simulink model "TargetModel"  (R2014a)
settings: Solver=ode3  SolverMode=SingleTasking  StartTime=0.0  StopTime=Inf  FixedStep=0.1  RelTol=1e-3
PostLoadFcn:
  | loadRobotParameters
  | 
  | allotedRunTime = 3*60; % [sec] Time allowed for run
  | 
  | % starting parameters
  | % The timer starts once the robot has moved a certain distance from the
  | % starting point
  | startPos = [50 50]; % [cm]
  | startingRadius = 10; % [cm]
  | 
  | % Target parameters
  | targetBoundaryRadius = 7; % [cm] radius considered at location
  | statTimeReq = 2.5; % [sec] minimum time robot must be at location
InitFcn:
  | close('all','force');
StartFcn:
  | %reset(SimDisplay.getInstance());
undefined symbols (not defined in the file or in its folder): AxleLength, dT, EncRes, TargetPositions, WheelRadius
libraries: arduinodue_drivers x5, simulink x3, arduinolib x2
CloseFcn:
  | close('all','force');
settings Model: SimulationMode=external  PauseTimes=14  ExtModeTrigDuration=2  Creator=gpacitti  LastModifiedBy=odufour
settings DataIOCC: SignalLoggingSaveFormat=ModelDataLogs  SaveOutput=off  SignalLogging=off  DSMLogging=off  SaveTime=off
settings OptimizationCC: ExpressionDepthLimit=2147483647  OptimizeModelRefInitCode=on  LifeSpan=Inf
settings DebuggingCC: UnderspecifiedInitializationDetection=Classic  SolverPrmCheckMsg=none  MultiTaskDSMMsg=warning  MultiTaskCondExecSysMsg=none  ParameterPrecisionLossMsg=none  StateNameClashWarn=warning
settings HardwareCC: ProdLargestAtomicInteger=Long  ProdLargestAtomicFloat=Double  ProdEndianess=LittleEndian  ProdHWDeviceType=ARM Compatible->ARM Cortex
settings RTWCC: SystemTargetFile=realtime.tlc  GenerateMakefile=off  TemplateMakefile=realtime.tmf  Description=Run on Target Hardware  RTWVerbose=off  ProcessScript=realtime_make_rtw_hook  IncludeERTFirstTime=on
settings CodeAppCC: CustomSymbolStrType=$N$R$M  InternalIdentifier=Classic
settings STFCustomTargetCC: TargetLibSuffix=.a  GenerateSampleERTMain=on  ConcurrentExecutionCompliant=off  GeneratePreprocessorConditionals=Use local settings  ERTCustomFileBanners=on  SupportNonInlinedSFcns=off  SupportVariableSizeSignals=on  MATLABClassNameForMDSCustomization=Simulink.SoftwareTarget.ERTCustomization  GRTInterface=off  SystemTargetFile=realtime.tlc
settings ERTTargetCC: CombineOutputUpdateFcns=off  SupportContinuousTime=on  SupportVariableSizeSignals=on  ExtMode=on  ExtModeTransport=3  ExtModeMexArgs=0 17 115200 30  ERTSrcFileBannerTemplate=realtime_code_template.cgt  ERTHdrFileBannerTemplate=realtime_code_template.cgt  ERTDataSrcFileTemplate=realtime_code_template.cgt  ERTDataHdrFileTemplate=realtime_code_template.cgt  ERTCustomFileTemplate=realtime_file_process.tlc
settings ConfigComp: Description=Design Verifier Custom Configuration Component  DVMaxTestCaseSteps=500  DVTestSuiteOptimization=CombinedObjectives (Nonlinear Extended)

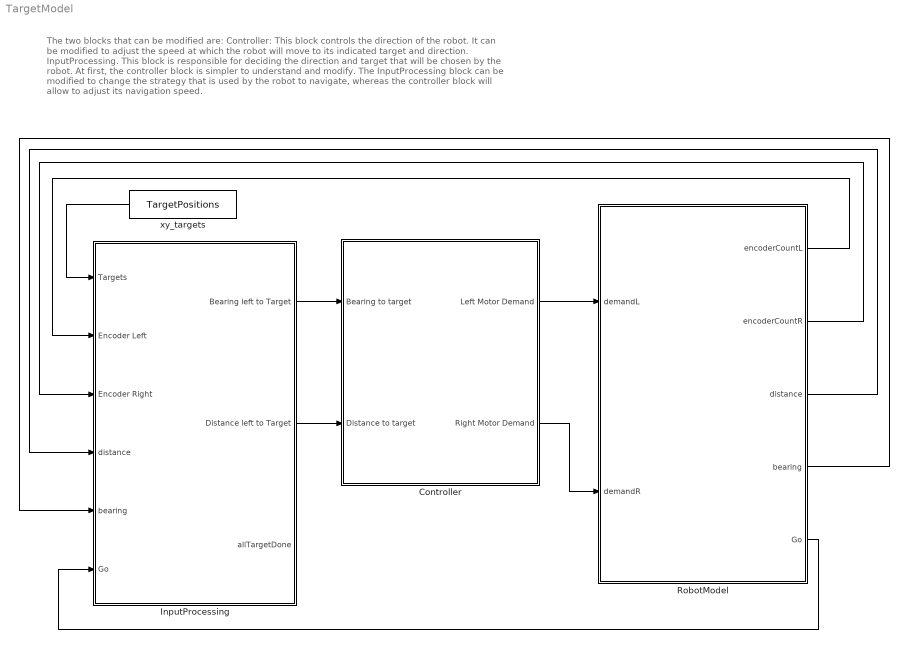
== system TargetModel ==
  note: The two blocks that can be modified are:
      | Controller: This block controls the direction of the robot. It can be modified to adjust the speed at which the robot will move to its indicated target and direction.
      | InputProcessing. This block is responsible for deciding the direction and target that will be chosen by the robot.
      |
      | At first, the controller block is simpler to understand and modify.
      | The InputProcessing block can be modified to change the strategy that is used by the robot to navigate, whereas the controller block will allow to adjust its navigation speed.
  Controller : Subsystem  TreatAsAtomicUnit=on
      mask Display: image('Arduino_Mega_2560.jpg',[0.75/2,0.3,0.25,0.4]);
  InputProcessing : Subsystem
      mask Display: image('Arduino_Mega_2560.jpg',[0.75/2,0.3,0.25,0.3]);
  RobotModel : Subsystem
      mask Display: image('robot_3d.jpg',[0.20,0.3,0.45,0.3]);
  xy_targets : Constant  Value=TargetPositions  OutDataTypeStr=single  SampleTime=1
  wires:
  RobotModel/2(encoderCountR) -> InputProcessing/3(Encoder Right)
  RobotModel/1(encoderCountL) -> InputProcessing/2(Encoder Left)
  xy_targets/1 -> InputProcessing/1(Targets)
  InputProcessing/2(Distance left to Target) -> Controller/2(Distance to target)
  InputProcessing/1(Bearing left to Target) -> Controller/1(Bearing to target)
  Controller/1(Left Motor Demand) -> RobotModel/1(demandL)
  Controller/2(Right Motor Demand) -> RobotModel/2(demandR)
  RobotModel/3(distance) -> InputProcessing/4(distance)
  RobotModel/4(bearing) -> InputProcessing/5(bearing)
  RobotModel/5(Go) -> InputProcessing/6(Go)

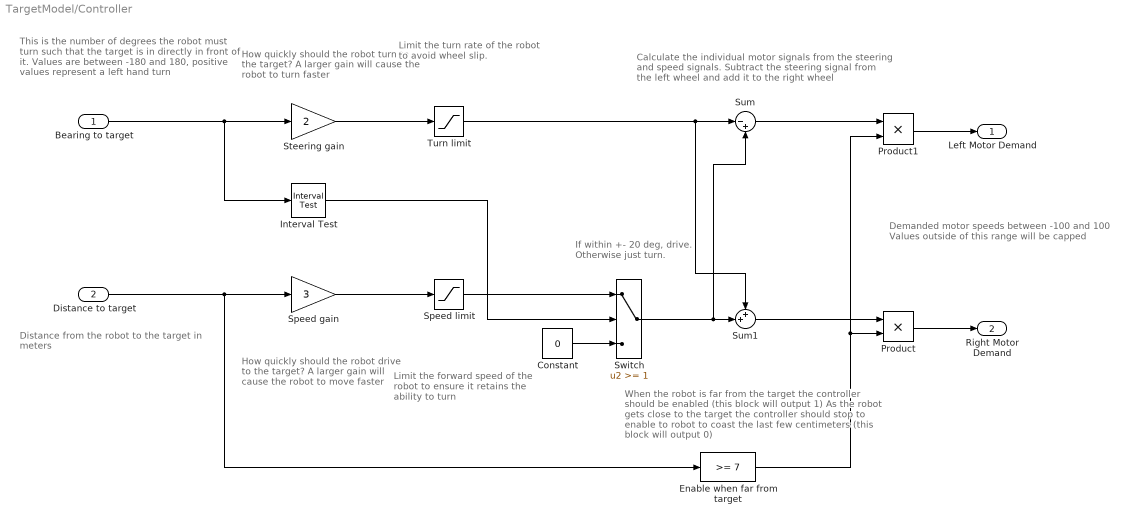
== system TargetModel/Controller ==
  note: This is the number of degrees the robot
      | must turn such that the target is in directly
      | in front of it.
      | Values are between -180 and 180,
      | positive values represent a left hand turn
  note: Distance from the robot to the target
      | in meters
  note: Demanded motor speeds between -100 and 100
      | Values outside of this range will be capped
  note: How quickly should the robot turn
      | to the target? A larger gain will
      |  cause the robot to turn faster
  note: How quickly should the robot
      | drive to the target? A larger gain
      | will cause the robot to move
      | faster
  note: Limit the forward speed of the
      | robot to ensure it retains the
      | ability to turn
  note: When the robot is far from the target the controller
      | should be enabled (this block will output 1)
      | As the robot gets close to the target the controller
      | should stop to enable to robot to coast the last
      | few centimeters (this block will output 0)
  note: Calculate the individual motor signals from the
      | steering and speed signals. Subtract the steering
      | signal from the left wheel and add it to the right
      | wheel
  note: If within +- 20 deg, drive.
      | Otherwise just turn.
  note: Limit the turn rate of the
      | robot to avoid wheel slip.
  Bearing to target : Inport  OutDataTypeStr=single
  Distance to target : Inport  Port=2  PortDimensions=1  SampleTime=dT
  Constant : Constant  Value=0  OutDataTypeStr=single
  Enable when far from target : simulink/Logic and Bit Operations/Compare To Constant  relop=>=  const=7  OutDataTypeStr=uint8
  Interval Test : simulink/Logic and Bit Operations/Interval Test  IntervalClosedRight=on  uplimit=20  IntervalClosedLeft=on  lowlimit=-20  OutDataTypeStr=boolean
      settings: AttributesFormatString=|
      | Upper = %<uplimit>
      | Lower = %<lowlimit>
  Product : Product
  Product1 : Product
  Speed gain : Gain  Gain=3
  Speed limit : Saturate  UpperLimit=40  LowerLimit=0
      settings: AttributesFormatString=|
      | Upper = %<UpperLimit>
      | Lower = %<LowerLimit>
  Steering gain : Gain  Gain=2
  Sum : Sum  Inputs=|-+
  Sum1 : Sum  Inputs=++|
  Switch : Switch  Threshold=1
  Turn limit : Saturate  UpperLimit=50  LowerLimit=-50
      settings: AttributesFormatString=|
      | Upper = %<UpperLimit>
      | Lower = %<LowerLimit>
  Left Motor Demand : Outport  OutDataTypeStr=single
  Right Motor Demand : Outport  Port=2  OutDataTypeStr=single
  wires:
  Speed limit/1 -> Switch/1
  Turn limit/1 -> Sum1/1, Sum/1
  Constant/1 -> Switch/3
  Interval Test/1 -> Switch/2
  Sum/1 -> Product1/1
  Sum1/1 -> Product/1
  Bearing to target/1 -> Steering gain/1, Interval Test/1
  Switch/1 -> Sum1/2, Sum/2
  Enable when far from target/1 -> Product1/2, Product/2
  Product1/1 -> Left Motor Demand/1
  Product/1 -> Right Motor Demand/1
  Speed gain/1 -> Speed limit/1
  Steering gain/1 -> Turn limit/1
  Distance to target/1 -> Enable when far from target/1, Speed gain/1

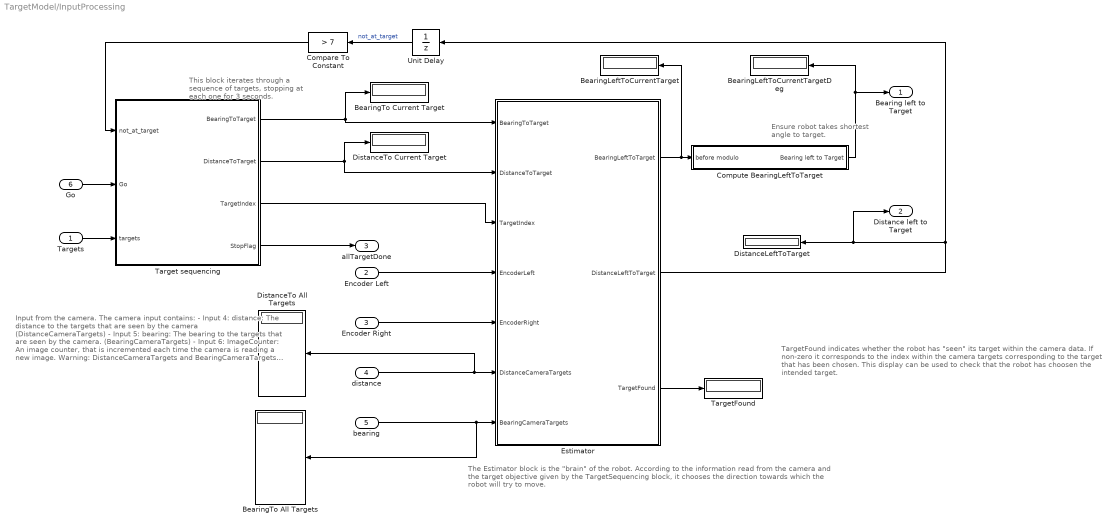
== system TargetModel/InputProcessing ==
  note: TargetFound indicates whether the robot has "seen" its target within the camera
      | data.
      | If non-zero it corresponds to the index within the camera targets corresponding
      | to the target that has been chosen.
      |
      | This display can be used to check that the robot has choosen the intended
      | target.
  note: The Estimator block is the "brain" of the robot. According to the information read from the camera and the
      | target objective given by the TargetSequencing block, it chooses the direction towards which the robot
      | will try to move.
  note: Ensure robot takes shortest
      | angle to target.
  note: This block iterates through a
      | sequence of targets, stopping
      | at each one for 3 seconds.
  note: Input from the camera. The camera input contains:
      | - Input 4: distance: The distance to the targets that are seen by the
      |   camera (DistanceCameraTargets)
      | - Input 5: bearing: The bearing to the targets that are seen
      |   by the camera. (BearingCameraTargets)
      | - Input 6: ImageCounter: An image counter, that is incremented
      |   each time the camera is reading a new image.
      | Warning: DistanceCameraTargets and BearingCameraTargets
      | are the targets seen by the camera. So for instance, the
      | target 1 is the first target seen by the camera, but is not the
      | same target as the target at index 1 within the target sequencing
      | block.
  Targets : Inport
  Encoder Left : Inport  Port=2  OutDataTypeStr=class(intEncoder(0))
  Encoder Right : Inport  Port=3  OutDataTypeStr=class(intEncoder(0))
  distance : Inport  Port=4
  bearing : Inport  Port=5
  Go : Inport  Port=6
  BearingLeftToCurrentTarget : Display
  BearingLeftToCurrentTargetDeg : Display
  BearingTo All Targets : Display
  "BearingTo Current Target " : Display
  Compare To Constant : simulink/Logic and Bit Operations/Compare To Constant  relop=>  const=7  OutDataTypeStr=boolean
  Compute BearingLeftToTarget : Subsystem
  DistanceLeftToTarget : Display
  DistanceTo All Targets : Display
  DistanceTo Current Target : Display
  Estimator : MATLAB Function  TreatAsAtomicUnit=on
  Target sequencing : MATLAB Function  TreatAsAtomicUnit=on  SystemSampleTime=dT
  TargetFound : Display
  Unit Delay : UnitDelay  SampleTime=dT
  Bearing left to Target : Outport  SampleTime=dT
  Distance left to Target : Outport  Port=2
  allTargetDone : Outport  Port=3
  wires:
  Go/1 -> Target sequencing/2(Go)
  distance/1 -> DistanceTo All Targets/1, Estimator/6(DistanceCameraTargets)
  bearing/1 -> Estimator/7(BearingCameraTargets), BearingTo All Targets/1
  Target sequencing/4(StopFlag) -> allTargetDone/1
  Compare To Constant/1 -> Target sequencing/1(not_at_target)
  Compute BearingLeftToTarget/1(Bearing left to Target) -> BearingLeftToCurrentTargetDeg/1, Bearing left to Target/1
  Estimator/3(TargetFound) -> TargetFound/1
  Target sequencing/3(TargetIndex) -> Estimator/3(TargetIndex)
  Estimator/2(DistanceLeftToTarget) -> DistanceLeftToTarget/1, Distance left to Target/1, Unit Delay/1
  Estimator/1(BearingLeftToTarget) -> BearingLeftToCurrentTarget/1, Compute BearingLeftToTarget/1(before modulo)
  Target sequencing/1(BearingToTarget) -> Estimator/1(BearingToTarget), "BearingTo Current Target "/1
  Unit Delay/1 -> Compare To Constant/1  "not_at_target"
  Encoder Right/1 -> Estimator/5(EncoderRight)
  Target sequencing/2(DistanceToTarget) -> Estimator/2(DistanceToTarget), DistanceTo Current Target/1
  Encoder Left/1 -> Estimator/4(EncoderLeft)
  Targets/1 -> Target sequencing/3(targets)

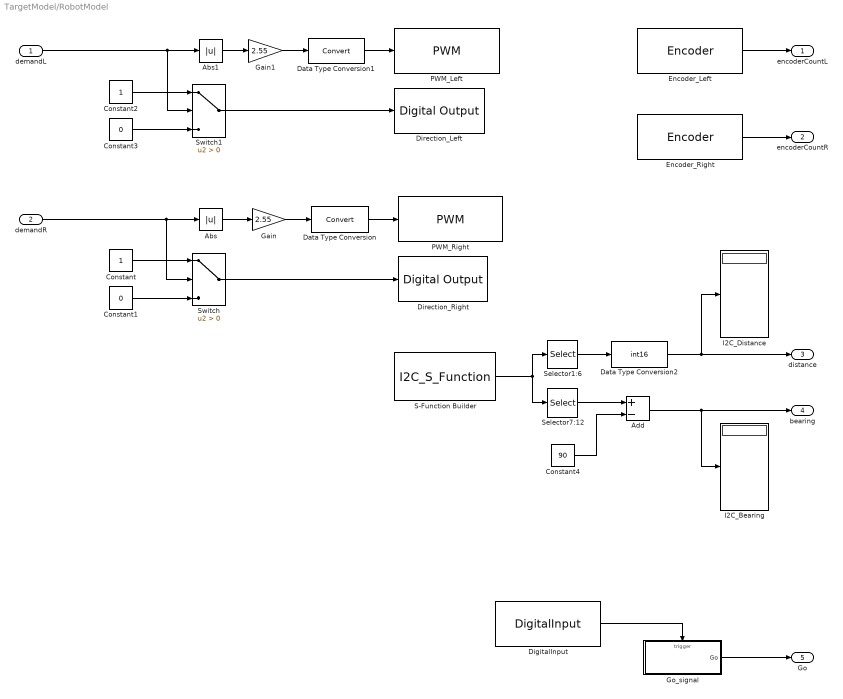
== system TargetModel/RobotModel ==
  demandL : Inport  SampleTime=0
  demandR : Inport  Port=2  SampleTime=0
  Abs : Abs
  Abs1 : Abs
  Add : Sum  Inputs=+-  OutDataTypeStr=int8
  Constant : Constant  OutDataTypeStr=uint8
  Constant1 : Constant  Value=0  OutDataTypeStr=uint8
  Constant2 : Constant  OutDataTypeStr=uint8
  Constant3 : Constant  Value=0  OutDataTypeStr=uint8
  Constant4 : Constant  Value=90  OutDataTypeStr=uint8
  Data Type Conversion : DataTypeConversion  SaturateOnIntegerOverflow=on
  Data Type Conversion1 : DataTypeConversion  SaturateOnIntegerOverflow=on
  Data Type Conversion2 : DataTypeConversion  OutDataTypeStr=int16  SaturateOnIntegerOverflow=on
  DigitalInput : arduinodue_drivers/DigitalInput  pinNumber=17  isPullUp=on
  Direction_Left : arduinolib/Digital Output  pinNumber=7
  Direction_Right : arduinolib/Digital Output  pinNumber=4
  Encoder_Left : arduinodue_drivers/Encoder  pinA=18  pinB=19
  Encoder_Right : arduinodue_drivers/Encoder  pinA=2  pinB=3
  Gain : Gain  Gain=2.55
  Gain1 : Gain  Gain=2.55
  Go_signal : Subsystem  TreatAsAtomicUnit=on
  I2C_Bearing : Display
  I2C_Distance : Display
  PWM_Left : arduinodue_drivers/PWM  pinNumber=6
  PWM_Right : arduinodue_drivers/PWM  pinNumber=5
  S-Function Builder : S-Function  InitFcn=try, set_param(gcb,'FunctionName','I2C_S_Function'), end  FunctionName=I2C_S_Function  Parameters=uint8(1)  SFunctionModules=I2C_S_Function_wrapper  EnableBusSupport=off  mask(S-Function Builder){}
      mask help: Simulink:masks:SFunctionBuilder_MD
      mask init:
      | val = [[.9  0.75 0.75 1 1 .9 .9 1]',[1 1 0.75 0.75 .9 .9 1 .9]'];try , sys = get_param(gcb,'SfunBuilderFcnName');if isempty(sys), sys = get_param(gcb,'FunctionName'); end,catch, sys = get_param(gcb,'FunctionName'); end
      settings: CopyFcn=set_param(gcbh,'LinkStatus','none')  PreSaveFcn=try, set_param(gcb,'FunctionName','I2C_S_Function'), end  OpenFcn=sfunctionwizard(gcbh)
      mask Display: plot(val(:,1),val(:,2)),disp(sys), port_label('input',1,'Send'), port_label('output',1,'Receive')
  Selector1:6 : Selector  InputPortWidth=12  Indices=[1:6]
  Selector7:12 : Selector  InputPortWidth=12  Indices=[7:12]
  Switch : Switch  Criteria=u2 > Threshold
  Switch1 : Switch  Criteria=u2 > Threshold
  encoderCountL : Outport  OutDataTypeStr=class(intEncoder(0))
  encoderCountR : Outport  Port=2  OutDataTypeStr=class(intEncoder(0))
  distance : Outport  Port=3
  bearing : Outport  Port=4
  Go : Outport  Port=5
  wires:
  Encoder_Right/1 -> encoderCountR/1
  Encoder_Left/1 -> encoderCountL/1
  Abs/1 -> Gain/1
  Gain/1 -> Data Type Conversion/1
  Data Type Conversion/1 -> PWM_Right/1
  Constant/1 -> Switch/1
  Constant1/1 -> Switch/3
  Switch/1 -> Direction_Right/1
  Abs1/1 -> Gain1/1
  Gain1/1 -> Data Type Conversion1/1
  Data Type Conversion1/1 -> PWM_Left/1
  Constant2/1 -> Switch1/1
  Constant3/1 -> Switch1/3
  Switch1/1 -> Direction_Left/1
  Data Type Conversion2/1 -> distance/1, I2C_Distance/1
  Add/1 -> I2C_Bearing/1, bearing/1
  demandR/1 -> Switch/2, Abs/1
  demandL/1 -> Switch1/2, Abs1/1
  DigitalInput/1 -> Go_signal/Trigger
  Go_signal/1(Go) -> Go/1
  S-Function Builder/1 -> Selector1:6/1, Selector7:12/1
  Selector7:12/1 -> Add/1
  Constant4/1 -> Add/2
  Selector1:6/1 -> Data Type Conversion2/1

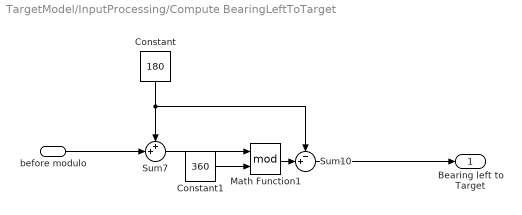
== system TargetModel/InputProcessing/Compute BearingLeftToTarget ==
  before modulo : Inport
  Constant : Constant  Value=180  OutDataTypeStr=Inherit: Inherit via back propagation
  Constant1 : Constant  Value=360  OutDataTypeStr=Inherit: Inherit via back propagation
  Math Function1 : Math  Operator=mod  SaturateOnIntegerOverflow=on
  Sum10 : Sum  Inputs=-+|
  Sum7 : Sum  Inputs=++|
  Bearing left to Target : Outport  SampleTime=dT
  wires:
  before modulo/1 -> Sum7/2
  Sum10/1 -> Bearing left to Target/1
  Math Function1/1 -> Sum10/2
  Constant1/1 -> Math Function1/2
  Sum7/1 -> Math Function1/1
  Constant/1 -> Sum10/1, Sum7/1

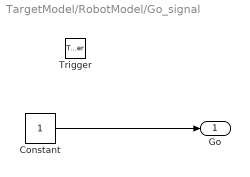
== system TargetModel/RobotModel/Go_signal ==
  Trigger : TriggerPort  TriggerType=falling
  Constant : Constant  OutDataTypeStr=uint8
  Go : Outport  OutDataTypeStr=uint8  InitialOutput=0
  wires:
  Constant/1 -> Go/1

== matlab function TargetModel/InputProcessing/Estimator ==
  data: BearingToTarget input; DistanceToTarget input; TargetIndex input; BearingLeftToTarget output; EncoderLeft input; DistanceLeftToTarget output; EncoderRight input; DistanceCameraTargets input; BearingCameraTargets input; TargetFound output; AxleLength parameter; WheelRadius parameter; EncRes parameter
function [BearingLeftToTarget, DistanceLeftToTarget, TargetFound] = ...
    estimator(BearingToTarget, DistanceToTarget, TargetIndex, EncoderLeft, ...
    EncoderRight, DistanceCameraTargets, BearingCameraTargets,...
    AxleLength, WheelRadius, EncRes)
%#codegen
%% This function computes the direction of the robot using:
% - The target that is selected by the target sequencer (i.e. the target
%   that the robot is intending to reach):
%   + BearingToTarget, DistanceToTarget, TargetIndex
% - The information from the wheel encoders:
%   + EncoderLeft (left wheel)
%   + EncoderRight (right wheel)
% - The information sent by the camera:
%   + DistanceCameraTargets: an array storing the distance to the camera
%     for each of the targets that are seen by the camera.
%   + BearingCameraTargets: an array storing the orientation to the 
%     target for each of the targets that are seen by the camera.
%   + ImageCounter: The acquisition counter from the camera: as the 
%     camera frequency is lower than the frequency of this block, this
%     block may be executed several time with the same information from
%     the camera.
%     ImageCounter can be used to indicate that the information is "fresh".


%% Index of the current target that the robot will try to reach.
% Storing it persistently allows us to determine when a new 
% target is selected
persistent  cur_target_index 

%% Values of the encoders left and right when reaching the
% last target.
persistent encoder_left_prev_target encoder_right_prev_target 

%% Those two variables are storing the position of the target 
% relative to the robot's position.
% They are updated when the robot is moving.
persistent distance_to_target bearing_to_target 
%% Stores the last image counter received from the camera. 
% It is used to check whether a new image has been received from the
% camera, since this block is executed more frequently than the camera.

if isempty(cur_target_index)
    %% Initializes the persistent values to default values
    cur_target_index = uint8(0);
    encoder_left_prev_target = int32(0);
    encoder_right_prev_target = int32(0);
    distance_to_target = single(0);
    bearing_to_target = single(0);
end

%% In the case where the target has changed, updates the target information.
if (cur_target_index ~= TargetIndex)
    cur_target_index = TargetIndex;
    % Save encoders value
    encoder_left_prev_target = EncoderLeft;
    encoder_right_prev_target = EncoderRight;
    bearing_to_target = BearingToTarget;
    distance_to_target = DistanceToTarget;
end

%%%%%%%%%%%%%%%%%%%%%
% Robot distance and angle based on encoders
% Axle length = 160mm
% Wheel diameter = 66.5mm
% Encoder = 12*53 = 636 ticks per wheel turn

%% Updates the position information from the encoders information.
dL = single(EncoderLeft - encoder_left_prev_target) * 2 * WheelRadius * pi / EncRes;
dR = single(EncoderRight - encoder_right_prev_target) * 2 * WheelRadius * pi / EncRes;
CurrentDistance = ((dL + dR)/2);
DistanceLeftToTarget = distance_to_target - CurrentDistance;

% Angle from prev target
CurrentBearing = single(((dR - dL)*180) / (AxleLength*pi));

BearingLeftToTarget = bearing_to_target - CurrentBearing;
% Ensure our robot angle stays within a single revolution
%BearingLeftToTarget = single(mod(BearingLeftToTarget,360));


%% Correction using the camera.
%
% In the case where a new image is received from the camera, 
% try to adjust the direction.
% This adjustment is only performed if the robot has traveled
% at least 5cm since the last target. This delay is here to 
% prevent changing the direction too often because of the
% camera input delay.
TargetFound=uint8(0);
dist_left = int16(DistanceLeftToTarget);
if(CurrentDistance > 5 && dist_left> 20 )
    %% Search for the target within the targets that are seen by the 
    % camera.
    % A target is chosen if it is at less than 10cms of the searched 
    % target, and within 36 degree.
    % In the case where several candidate targets are seen, the target
    % chosen is the target that is the closest to the expected distance.
    for ind=1:length(DistanceCameraTargets)
        if(DistanceCameraTargets(ind) > 5 )
            if(abs(DistanceCameraTargets(ind) - dist_left)<10 && ...
                    abs(BearingCameraTargets(ind))<36 )
                if (TargetFound==0 || abs(DistanceCameraTargets(TargetFound) - ...
                        dist_left)>abs(DistanceCameraTargets(ind) - dist_left))
                    TargetFound=uint8(ind);
                end
            end
        end
    end

    if ( TargetFound ~= 0)
        %% In the case where a target has been found, adjust the 
        % information.
        DistanceLeftToTarget = single(DistanceCameraTargets(TargetFound));   % data from camera
        BearingLeftToTarget = single(BearingCameraTargets(TargetFound))/2;   % data from camera
        % Reset encoders
        encoder_left_prev_target = EncoderLeft;
        encoder_right_prev_target = EncoderRight;
        bearing_to_target = BearingLeftToTarget;
        distance_to_target = DistanceLeftToTarget;
    else
        %% Not target found.
        % TODO: This code could be removed (TargetFound is already 0), but
        TargetFound=uint8(0);
        DistanceLeftToTarget=DistanceLeftToTarget;  %#ok<ASGSL> data from encoders
        BearingLeftToTarget=BearingLeftToTarget;    %#ok<ASGSL> data from encoders
    end
end

== matlab function TargetModel/InputProcessing/Target sequencing ==
  data: not_at_target input boolean; Go input; BearingToTarget output single; targets input single; DistanceToTarget output; TargetIndex output uint8; StopFlag output boolean
function [BearingToTarget,DistanceToTarget,TargetIndex,StopFlag]= sequencer(not_at_target,Go,targets)
%#codegen

%% This block is chosing target that the robot will try to reach.
% It returns the direction and distance to the next target from the 
% previous target (i.e. the direction and distance are not adjusted
% when the robot is moving).
% Its inputs are:
% - not_at_target: indicates whether the robot is on a target or not.
% - targets: the list of targets, in the order that they will be 
%   reached.
% Its outputs are:
% - BearingToTarget: The bearing to the next target, from the previous 
%   target.
% - DistanceToTarget: The distance to the next target, from the previous
%   target.
% - TargetIndex: the index of the target.
% - StopFlag: set to true when the robot has moved through all the targets.


% The time in seconds the robot will wait when it reaches a target before
% selecting the new target.
pause_time = single(3);

% Persistent variables are used to store the internal state of the block:
% - target_index: The index of the current target.
% - wait_timer: Timer that is used to pause at the targets
% - stop_flag: Set to true when all the targets have been reached.
% - prev_target: The previous target.
% - prev_bearing: The previous bearing
% - distance_to_target: The distance_to the next target (from the previous
%   target).
% - bearing_to_target: The bearing to the next target (from the expected 
%   orientation when reaching the previous target).
persistent target_index wait_timer stop_flag prev_target prev_bearing distance_to_target bearing_to_target

if isempty(target_index)
    %% Initializes persistent variables to the default state
    target_index = uint8(0);
    wait_timer = single(0);
    stop_flag = false;
    prev_target = single([ 50; 50 ]);
    prev_bearing = single(0);
    distance_to_target = single(0);
    bearing_to_target = single(0);
end

%% Computation of the target sequencing:
%  - If the target is not reached, the wait timer is reset to the 
%    pause time.
%  - If the target is reached, the wait timer is decremented, and 
%    a new target is selected when it reaches zero.
if not_at_target || ~Go
    wait_timer = pause_time;
else
    wait_timer = wait_timer - 0.1;
    if wait_timer <= 0
        %% At target, and time elapsed. Reset timer, and computes
        % bearing and orientation to the target.
        wait_timer = pause_time;
        if target_index < length(targets)
            % Next target
            target_index = target_index + 1;
            current_target_pos = [targets(target_index,1);targets(target_index,2)];
            distance_to_target = (norm(current_target_pos-prev_target));
            dy = current_target_pos(2)-prev_target(2);
            dx = current_target_pos(1)-prev_target(1);
            bearing_to_target = (atan2d(dy,dx));
            bearing_to_target = bearing_to_target-prev_bearing;
            prev_target=[targets(target_index,1);targets(target_index,2)];
            prev_bearing=prev_bearing+bearing_to_target;
        else
            wait_timer = pause_time;
            stop_flag = true;
        end
    end    
end

%% Sets the output from the previously computed values.
DistanceToTarget = distance_to_target;
BearingToTarget = bearing_to_target;
TargetIndex = target_index;
StopFlag = stop_flag ;
